simulink model "model"  (R2019a)
settings: Solver=VariableStepAuto  StartTime=0.0  StopTime=10.0  RelTol=1e-3
undefined symbols (not defined in the file or in its folder): init_states, l_f, l_r, v_angle
settings Model: Creator=jacoboffersen  LastModifiedBy=jacoboffersen

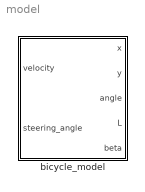
== system model ==
  "bicycle_model " : Subsystem

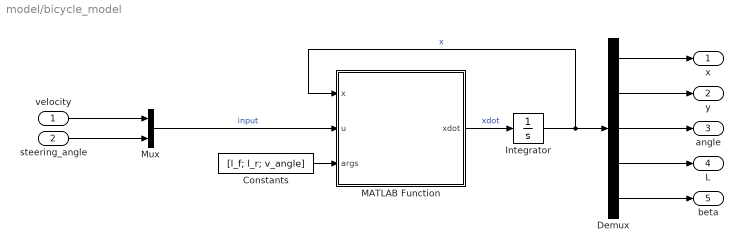
== system model/bicycle_model  ==
  velocity : Inport
  "steering_angle " : Inport  Port=2
  Constants : Constant  Value=[l_f; l_r; v_angle]
  Demux : Demux  Outputs=5
  Integrator : Integrator  InitialCondition=[init_states;0]
  MATLAB Function : MATLAB Function  TreatAsAtomicUnit=on
  Mux : Mux  Inputs=2
  x : Outport
  y : Outport  Port=2
  angle : Outport  Port=3
  L : Outport  Port=4
  beta : Outport  Port=5
  wires:
  Mux/1 -> MATLAB Function/2(u)  "input"
  velocity/1 -> Mux/1
  "steering_angle "/1 -> Mux/2
  Constants/1 -> MATLAB Function/3(args)
  MATLAB Function/1(xdot) -> Integrator/1  "xdot"
  Integrator/1 -> MATLAB Function/1(x), Demux/1  "x"
  Demux/1 -> x/1
  Demux/2 -> y/1
  Demux/3 -> angle/1
  Demux/4 -> L/1
  Demux/5 -> beta/1

== matlab function model/bicycle_model /MATLAB Function ==
  data: x input; xdot output; u input; args input
function xdot = fcn(x, u, args)

x_pos            = x(1); % x pos
y_pos            = x(2); % y pos
yaw_angle        = x(3); % Yaw angle

velocity         = u(1); % Velocity
steering_angle   = u(2); % Steering angle

length_front     = args(1); % Length from front axle to CG
length_rear      = args(2); % Length fromt rear axle to CG
velocity_angle   = args(3); % Angle of velocity

slip_angle = atan(length_rear * tan(steering_angle) / (length_front + length_rear));

x_change = velocity * cos(yaw_angle + slip_angle);
y_change = velocity * sin(yaw_angle + slip_angle);
L_change = x_change * sin(velocity_angle) + y_change * cos(velocity_angle);
yaw_rate = tan(ster_ang) * velocity * cos(slip_angle)/(length_front + length_rear);

xdot = [x_change; y_change; yaw_rate; L_change; slip_angle];
